simulink library "mbd_s32k11_ec_toolbox"  (Simulink 9.0)
settings: Solver=FixedStepDiscrete  StartTime=0.0  StopTime=10.0  FixedStep=0.1  RelTol=1e-3
InitFcn:
  | mbd_s32k11_consistency_checks(bdroot(gcs));
(part 2 of 2)

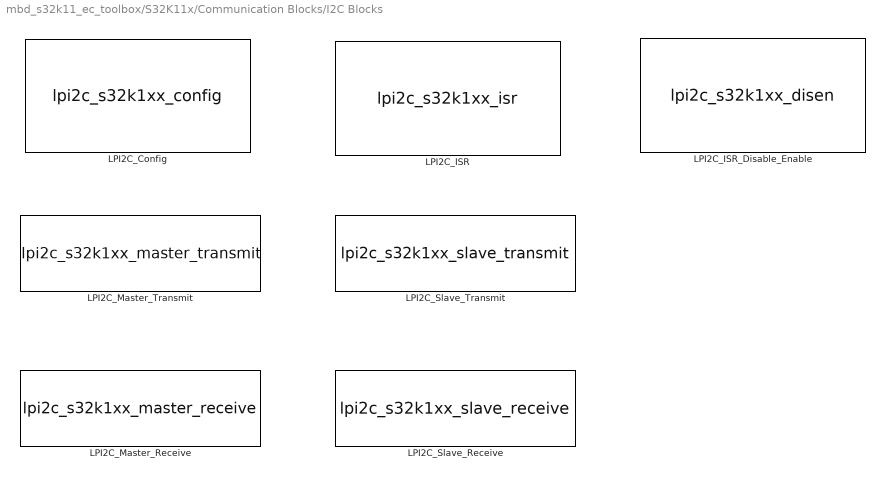
== system mbd_s32k11_ec_toolbox/S32K11x/Communication Blocks/I2C Blocks ==
  LPI2C_Config : S-Function  FunctionName=lpi2c_s32k1xx_config  SFunctionDeploymentMode=off  EnableBusSupport=off  mask(lpi2c_s32k1xx_config){instance=0, mode=Master, opmode=Standard (up to 100 kbit/s), bdr=100000, addr=1, is10bitaddr=off, sda=PTA2: [LPI2C0_SDA | LPI2C Data I/O], scl=PTA3: [LPI2C0_SCL | LPI2C Clock I/O]}
      mask prompts: opmode "Operating mode"; bdr "Baudrate, b/s"; addr "null"; is10bitaddr "10-bit address"
      mask help: This block allows to configure I2C module.
      mask init:
      | maskStr = mbd_s32k_lpi2c_config_string();
      | mbd_s32k_lpi2c_display_instances();
      | mbd_s32k_lpi2c_instance_callback(gcb);
      settings: NameChangeFcn=mbd_s32k_name_check(gcb);
      mask Help: web(fullfile(mbd_s32k11_block_help, 'lpi2c', 'lpi2c_config.html'));
      mask TypeOptions instance: 0
      mask Callback instance:
      | mbd_s32k_lpi2c_instance_callback(gcb);
      | mbd_s32k_lpi2c_display_instances();
      mask TypeOptions mode: Master | Slave
      mask Callback mode: mbd_s32k_lpi2c_mode_callback(gcb);
      mask TypeOptions opmode: Standard (up to 100 kbit/s)
      mask Callback bdr: mbd_s32k_lpi2c_check_bdr(gcb);
      mask TypeOptions sda: PTA2: [LPI2C0_SDA | LPI2C Data I/O] | PTB6: [LPI2C0_SDA | LPI2C Data I/O]
      mask TypeOptions scl: PTA3: [LPI2C0_SCL | LPI2C Clock I/O] | PTB7: [LPI2C0_SCL | LPI2C Clock I/O]
      mask Display: disp(maskStr);
  LPI2C_ISR : S-Function  FunctionName=lpi2c_s32k1xx_isr  SFunctionDeploymentMode=off  EnableBusSupport=off  mask(lpi2c_s32k1xx_isr){instance=0, mode=Master, rxreq=off, txreq=off, txempty=off, rxfull=off, stop=off, masterendtransfer=off, mastertx=off, masterrx=off, masterfifoerr=off, masterarblost=off, masternack=off}
      mask prompts: rxreq "I2C_SLAVE_EVENT_RX_REQ"; txreq "I2C_SLAVE_EVENT_TX_REQ"; txempty "I2C_SLAVE_EVENT_TX_EMPTY"; rxfull "I2C_SLAVE_EVENT_RX_FULL"; stop "I2C_SLAVE_EVENT_STOP"; masterendtransfer "I2C_MASTER_EVENT_END_TRANSFER"; mastertx "LPI2C_MASTER_EVENT_TX"; masterrx "LPI2C_MASTER_EVENT_RX"; masterfifoerr "LPI2C_MASTER_EVENT_FIFO_ERROR"; masterarblost "LPI2C_MASTER_EVENT_ARBITRATION_LOST"; masternack "LPI2C_MASTER_EVENT_NACK"
      mask help: This block allows to create routine for the LPI2C interrupts.
      mask init:
      | st = mbd_s32k_lpi2c_isr_tostring();
      | mbd_s32k_lpi2c_display_instances();
      settings: NameChangeFcn=mbd_s32k_name_check(gcb);
      mask Help: web(fullfile(mbd_s32k11_block_help, 'lpi2c', 'lpi2c_isr.html'));
      mask TypeOptions instance: 0
      mask Callback instance: mbd_s32k_lpi2c_display_instances();
      mask TypeOptions mode: Master | Slave
      mask Callback mode: mbd_s32k_lpi2c_isr_mode_ckb(gcb);
      mask Display:
      | disp(st);
      | port_label('output', 1, 'Trigger')
  LPI2C_ISR_Disable_Enable : S-Function  FunctionName=lpi2c_s32k1xx_disen  SFunctionDeploymentMode=off  EnableBusSupport=off  mask(lpi2c_s32k1xx_disen){instance=0, m_tdie=off, m_rdie=off, m_epie=off, m_sdie=off, m_ndie=off, m_alie=off, m_feie=off, s_tdie=off, s_rdie=off, s_rsie=off, s_sdie=off, s_beie=off, s_feie=off, upd=1}
      mask prompts: m_tdie "Transmit Data"; m_rdie "Receive Data"; m_epie "End Packet"; m_sdie "STOP Detect"; m_ndie "NACK Detect"; m_alie "Arbitration Lost"; m_feie "FIFO Error"; s_tdie "Transmit Data"; s_rdie "Receive Data"; s_rsie "Repeated Start"; s_sdie "STOP Detect"; s_beie "Bit Error"; s_feie "FIFO Error"
      mask help: This block allows to Enable/Disable I2C ISR routine.
      mask init:
      | mbd_s32k_lpi2c_display_instances();
      | 
      | eol = sprintf('\n');
      | st = ['LPI2C', get_param(gcb, 'instance')];
      | fields = get_param(gcb, 'MaskPrompts');
      | vis = get_param(gcb, 'MaskVisibilities');
      | vals = get_param(gcb, 'MaskValues');
      | 
      | for i = 2 : length(fields) - 1
      |     if (strcmp(vis{i}, 'on'))
      |         s = [eol, fields{i}, ': ', vals{i}];
      |         st = [st, s];
      |     end
      | end
      settings: NameChangeFcn=mbd_s32k_name_check(gcb);
      mask Help: web(fullfile(mbd_s32k11_block_help, 'lpi2c', 'lpi2c_disen.html'));
      mask TypeOptions instance: 0
      mask Callback instance: mbd_s32k_lpi2c_display_instances();
      mask Display: disp(st);
  LPI2C_Master_Receive : S-Function  FunctionName=lpi2c_s32k1xx_master_receive  SFunctionDeploymentMode=off  EnableBusSupport=off  mask(lpi2c_master_receive){instance=0, xfermode=Blocking, Timeout=50, is10bit=off}
      mask prompts: xfermode "Transfer mode"; Timeout "Timeout (ms)"; is10bit "10-bit address"
      mask help: This block allows the master to request data from slave.
      mask init:
      | maskStr = 'LPI2C Master Receive';
      | mbd_s32k_lpi2c_display_instances();
      settings: NameChangeFcn=mbd_s32k_name_check(gcb);
      mask Help: web(fullfile(mbd_s32k11_block_help, 'lpi2c', 'lpi2c_master_receive.html'));
      mask TypeOptions instance: 0
      mask Callback instance: mbd_s32k_lpi2c_display_instances();
      mask TypeOptions xfermode: Blocking | Non blocking
      mask Callback xfermode: mbd_s32k_lpi2c_xfer_mode_cbk()
      mask Display:
      | port_label('output', 1, 'Data');
      | port_label('input', 1, 'Address');
      | port_label('input', 2, 'SendStop');
      | port_label('input', 3, 'Length');
      | disp(maskStr);
  LPI2C_Master_Transmit : S-Function  FunctionName=lpi2c_s32k1xx_master_transmit  SFunctionDeploymentMode=off  EnableBusSupport=off  mask(lpi2c_master_transmit){instance=0, xfermode=Blocking, Timeout=50, is10bit=off}
      mask prompts: xfermode "Transfer mode"; Timeout "Timeout (ms)"; is10bit "10-bit address"
      mask help: This block allows the master to transmit data to the slave.
      mask init:
      | maskStr = 'LPI2C Master Transmit';
      | mbd_s32k_lpi2c_display_instances();
      settings: NameChangeFcn=mbd_s32k_name_check(gcb);
      mask Help: web(fullfile(mbd_s32k11_block_help, 'lpi2c', 'lpi2c_master_transmit.html'));
      mask TypeOptions instance: 0
      mask Callback instance: mbd_s32k_lpi2c_display_instances();
      mask TypeOptions xfermode: Blocking | Non blocking
      mask Callback xfermode: mbd_s32k_lpi2c_xfer_mode_cbk()
      mask Display:
      | port_label('input', 1, 'Data');
      | port_label('input', 2, 'SendStop');
      | port_label('input', 3, 'Address');
      | disp(maskStr);
  LPI2C_Slave_Receive : S-Function  FunctionName=lpi2c_s32k1xx_slave_receive  SFunctionDeploymentMode=off  EnableBusSupport=off  mask(lpi2c_slave_receive){instance=0, xfermode=Blocking, Timeout=50, is10bit=off}
      mask prompts: xfermode "Transfer mode"; Timeout "Timeout (ms)"; is10bit "10-bit address"
      mask help: This block allows the slave to receive data from master.
      mask init:
      | maskStr = 'LPI2C Slave Receive';
      | mbd_s32k_lpi2c_display_instances();
      settings: NameChangeFcn=mbd_s32k_name_check(gcb);
      mask Help: web(fullfile(mbd_s32k11_block_help, 'lpi2c', 'lpi2c_slave_receive.html'));
      mask TypeOptions instance: 0
      mask Callback instance: mbd_s32k_lpi2c_display_instances();
      mask TypeOptions xfermode: Blocking | Non blocking
      mask Callback xfermode: mbd_s32k_lpi2c_xfer_mode_cbk()
      mask Display:
      | port_label('output', 1, 'Data');
      | port_label('input', 1, 'Address');
      | port_label('input', 2, 'Length');
      | disp(maskStr);
  LPI2C_Slave_Transmit : S-Function  FunctionName=lpi2c_s32k1xx_slave_transmit  SFunctionDeploymentMode=off  EnableBusSupport=off  mask(lpi2c_slave_transmit){instance=0, xfermode=Blocking, Timeout=50, is10bit=off}
      mask prompts: xfermode "Transfer mode"; Timeout "Timeout (ms)"; is10bit "10-bit address"
      mask help: This block allows the slave to respond to master request for data.
      mask init:
      | maskStr = 'LPI2C Slave Transmit';
      | mbd_s32k_lpi2c_display_instances();
      settings: NameChangeFcn=mbd_s32k_name_check(gcb);
      mask Help: web(fullfile(mbd_s32k11_block_help, 'lpi2c', 'lpi2c_slave_transmit.html'));
      mask TypeOptions instance: 0
      mask Callback instance: mbd_s32k_lpi2c_display_instances();
      mask TypeOptions xfermode: Blocking | Non blocking
      mask Callback xfermode: mbd_s32k_lpi2c_xfer_mode_cbk()
      mask Display:
      | port_label('input', 1, 'Data');
      | port_label('input', 2, 'Address');
      | disp(maskStr);

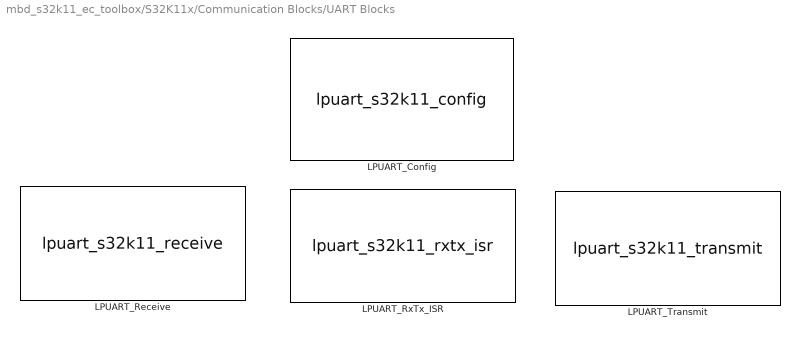
== system mbd_s32k11_ec_toolbox/S32K11x/Communication Blocks/UART Blocks ==
  LPUART_Config : S-Function  FunctionName=lpuart_s32k11_config  SFunctionDeploymentMode=off  EnableBusSupport=off  mask(lpuart_s32k11_config){instance=0, baudrate=115200, databits=8, parity=None, sbns=1, bothedge=rising edge, rxinv=off, txinv=off, show_adv_opts=off, brk13=10 - 13 bit times, lbkde=10 - 13 bit times, rx=PTA2: [LPUART0_RX | Receive], tx=PTA3: [LPUART0_TX | Transmit], cts=PTA0: [LPUART0_CTS | Clear To Send (bar)], rts=PTA1: [LPUART0_RTS | Request To Send]}
      mask prompts: instance "LPUART"; baudrate "Baud rate"; databits "Data bits"; parity "Parity mode"; sbns "Stop bit number select"; bothedge "Both edge sampling"; rxinv "Receive data inversion"; txinv "Transmit data inversion"; show_adv_opts "Show advanced options"; brk13 "Transmit break character length"; lbkde "Receive break character detection length"
      mask help: This block allows to configure LPUART module.
      mask init:
      | maskStr = mbd_s32k_lpuart_config_init();
      | mbd_s32k_lpuart_display_instances();
      | mbd_s32k_lpuart_instance_callback(gcb);
      settings: NameChangeFcn=mbd_s32k_name_check(gcb);
      mask Help: web(fullfile(mbd_s32k11_block_help, 'lpuart', 'lpuart_config.html'));
      mask TypeOptions instance: 0 | 1
      mask Callback instance:
      | mbd_s32k_lpuart_instance_callback(gcb);
      | mbd_s32k_lpuart_display_instances();
      mask TypeOptions baudrate: 1200 | 2400 | 4800 | 9600 | 14400 | 19200 | 38400 | 56000 | 57600 | 115200 | 128000 | 256000
      mask TypeOptions databits: 8 | 9 | 10
      mask TypeOptions parity: None | Even | Odd
      mask TypeOptions sbns: 1 | 2
      mask TypeOptions bothedge: rising edge | rising and falling edges
      mask Callback show_adv_opts: mbd_s32k_lpuart_config_cbk()
      mask TypeOptions brk13: 10 - 13 bit times | 13 - 16 bit times
      mask TypeOptions lbkde: 10 - 13 bit times | 13 - 16 bit times
      mask TypeOptions rx: PTA2: [LPUART0_RX | Receive] | PTB0: [LPUART0_RX | Receive] | PTC2: [LPUART0_RX | Receive]
      mask TypeOptions tx: PTA3: [LPUART0_TX | Transmit] | PTB1: [LPUART0_TX | Transmit] | PTC3: [LPUART0_TX | Transmit]
      mask TypeOptions cts: PTA0: [LPUART0_CTS | Clear To Send (bar)] | PTC8: [LPUART0_CTS | Clear To Send (bar)]
      mask TypeOptions rts: PTA1: [LPUART0_RTS | Request To Send] | PTC9: [LPUART0_RTS | Request To Send]
      mask Display: disp(maskStr);
  LPUART_Receive : S-Function  FunctionName=lpuart_s32k11_receive  SFunctionDeploymentMode=off  EnableBusSupport=off  mask(lpuart_s32k11_receive){instance=0}
      mask prompts: instance "LPUART"
      mask help: This block allows to read data from LPUART.
      mask init:
      | mbd_s32k_lpuart_display_instances();
      settings: NameChangeFcn=mbd_s32k_name_check(gcb);
      mask Help: web(fullfile(mbd_s32k11_block_help, 'lpuart', 'lpuart_receive.html'));
      mask TypeOptions instance: 0 | 1
      mask Callback instance: mbd_s32k_lpuart_display_instances();
      mask Display:
      | disp(['LPUART', get_param(gcb, 'instance')]);
      | port_label('output',1,'data');
      | port_label('input',1,'size');
  LPUART_RxTx_ISR : S-Function  FunctionName=lpuart_s32k11_rxtx_isr  Parameters=out_array  SFunctionDeploymentMode=off  EnableBusSupport=off  mask(lpuart_s32k11_rxtx_isr){instance=0, prio=0, tie=off, tcie=off, rie=off, ilie=off}
      mask prompts: instance "LPUART"; prio "ISR Priority"; tie "Transmit buffer empty"; tcie "End of transfer"; rie "Receiver buffer full"; ilie "Error event"
      mask help: This block allows to create receive/transmit ISR routine for the LPUART module.
      mask init:
      | mbd_s32k_lpuart_display_instances();
      | [out_struct, out_array] = mbd_s32k_lpuart_isr_info(gcb);
      | maskStr = mbd_s32k_lpuart_isr_string();
      settings: NameChangeFcn=mbd_s32k_name_check(gcb);
      mask Help: web(fullfile(mbd_s32k11_block_help, 'lpuart', 'lpuart_rxtx_isr.html'));
      mask TypeOptions instance: 0 | 1
      mask Callback instance: mbd_s32k_lpuart_display_instances();
      mask TypeOptions prio: 0 | 1 | 2 | 3 | 4 | 5 | 6 | 7 | 8 | 9 | 10 | 11 | 12 | 13 | 14 | 15
      mask Display:
      | port_label('output',1,'Trigger')
      | port_label('output',2,'Status')
      | disp(maskStr);
  LPUART_Transmit : S-Function  FunctionName=lpuart_s32k11_transmit  SFunctionDeploymentMode=off  EnableBusSupport=off  mask(lpuart_s32k11_transmit){instance=0}
      mask prompts: instance "LPUART"
      mask help: This block allows to transmit data via LPUART.
      mask init:
      | mbd_s32k_lpuart_display_instances();
      settings: NameChangeFcn=mbd_s32k_name_check(gcb);
      mask Help: web(fullfile(mbd_s32k11_block_help, 'lpuart', 'lpuart_transmit.html'));
      mask TypeOptions instance: 0 | 1
      mask Callback instance: mbd_s32k_lpuart_display_instances();
      mask Display:
      | disp(['LPUART', get_param(gcb, 'instance')]);
      | port_label('input',1,'data')

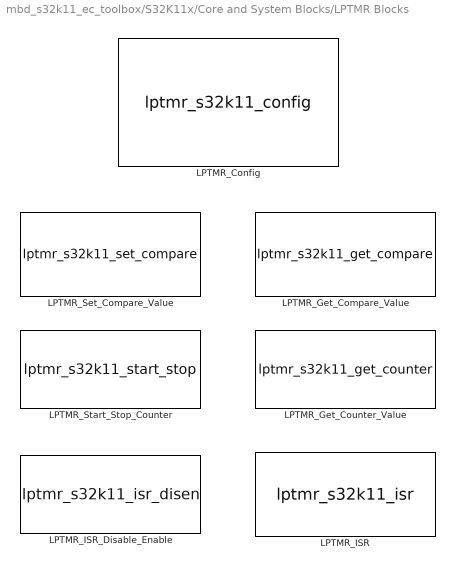
== system mbd_s32k11_ec_toolbox/S32K11x/Core and System Blocks/LPTMR Blocks ==
  LPTMR_Config : S-Function  FunctionName=lptmr_s32k11_config  SFunctionDeploymentMode=off  EnableBusSupport=off  mask(lptmr_s32k11_config){work_mode=Time Counter mode, compare_value=1, compare_value_units=Ticks, pin_select=Count pulses from pin alternative 2, pin_polarity=Count pulse on rising edge, pin_trgmux_source=Trigger function is disabled, show_adv_opts=off, input_clock=SIRC DIV2 clock, prescaler=Timer mode: prescaler 2, Glitch filter mode: invalid, bypass_prescaler=off, free_run=off, start_counter=on, enable_isr=on}
      mask prompts: work_mode "Mode Select"; compare_value "Compare Value"; compare_value_units "Compare Value Units"; pin_select "Pin Select"; pin_polarity "Pin Polarity"; pin_trgmux_source "TRGMUX Source"; show_adv_opts "Show advanced options"; input_clock "Prescaler Clock Select"; prescaler "Prescale Value"; bypass_prescaler "Prescaler Bypass"; free_run "Timer Free-Running Counter"; start_counter "Start  LPTMR counter immediatly after initialization"; enable_isr "Enable ISR immediatly after initialization"
      mask help: This block allows the user to configure the LPTMR module.
      mask init:
      | maskStr = mbd_s32k_lptmr_init();
      | 
      | set_param(gcb, 'MaskDisplay', ['disp(maskStr);']);
      settings: NameChangeFcn=mbd_s32k_name_check(gcb);
      mask Help: web(fullfile(mbd_s32k11_block_help, 'lptmr', 'lptmr_config.html'));
      mask TypeOptions work_mode: Time Counter mode | Pulse Counter mode
      mask Callback work_mode: mbd_s32k_lptmr_config_cbk('mode')
      mask TypeOptions compare_value_units: Ticks | Microseconds
      mask Callback compare_value_units: mbd_s32k_lptmr_config_cbk('units')
      mask TypeOptions pin_select: Count pulses from pin alternative 2 | Count pulses from pin alternative 3 | Count pulses from TRGMUX trigger
      mask Callback pin_select: mbd_s32k_lptmr_config_cbk('trgmux')
      mask TypeOptions pin_polarity: Count pulse on rising edge | Count pulse on falling edge
      mask TypeOptions pin_trgmux_source: Trigger function is disabled | Trigger MUX input 0 | Trigger MUX input 1 | Trigger MUX input 2 | Trigger MUX input 3 | Trigger MUX input 4 | Trigger MUX input 5 | Trigger MUX input 6 | Trigger MUX input 7 | Trigger MUX input 8 | Trigger MUX input 9 | Trigger MUX input 10 | Trigger MUX input 11 | CMP0 Output | LPIT Channel 0 | LPIT Channel 1 | LPIT Channel 2 | LPIT Channel 3 | LPTMR0 Trigger | FTM0 Internal Trigger | FTM0 External Trigger | FTM1 Internal Trigger | FTM1 External Trigger | FTM2 Internal Trigger | FTM2 External Trigger | FTM3 Internal Trigger | FTM3 External Trigger | ADC0_COCOA | ADC0_COCOB | ADC1_COCOA | ADC1_COCOB | PDB0 Channel 0 Trigger | PDB0 Pulse out | PDB1 Channel 0 Trigger | PDB1 Pulse out | RTC Alarm | RTC Seconds Counter | Flex IO Trigger 0 | Flex IO Trigger 1 | Flex IO Trigger 2 | Flex IO Trigger 3 | LPUART0 RX Data | LPUART0 TX Data | LPUART0 RX Idle | LPUART1 RX Data | LPUART1 TX Data | LPUART1 RX Idle | LPI2C0 Master Stop | LPI2C0 Slave Stop | LPI2C1 Master Stop | LPI2C1 Slave Stop | LPSPI0 Frame | LPSPI0 RX Data | LPSPI1 Frame | LPSPI1 RX Data | SIM Software Trigger
      mask Callback show_adv_opts: mbd_s32k_lptmr_config_cbk('show_adv_opts')
      mask TypeOptions input_clock: SIRC DIV2 clock | 1kHz LPO clock | RTC clock | PCC configured clock
      mask TypeOptions prescaler: Timer mode: prescaler 2, Glitch filter mode: invalid | Timer mode: prescaler 4, Glitch filter mode: 2 clocks | Timer mode: prescaler 8, Glitch filter mode: 4 clocks | Timer mode: prescaler 16, Glitch filter mode: 8 clocks | Timer mode: prescaler 32, Glitch filter mode: 16 clocks | Timer mode: prescaler 64, Glitch filter mode: 32 clocks | Timer mode: prescaler 128, Glitch filter mode: 64 clocks | Timer mode: prescaler 256, Glitch filter mode: 128 clocks | Timer mode: prescaler 512, Glitch filter mode: 256 clocks | Timer mode: prescaler 1024, Glitch filter mode: 512 clocks | Timer mode: prescaler 2048, Glitch filter mode: 1024 clocks | Timer mode: prescaler 4096, Glitch filter mode: 2048 clocks | Timer mode: prescaler 8192, Glitch filter mode: 4096 clocks | Timer mode: prescaler 16384, Glitch filter mode: 8192 clocks | Timer mode: prescaler 32768, Glitch filter mode: 16384 clocks | Timer mode: prescaler 65536, Glitch filter mode: 32768 clocks
      mask Callback bypass_prescaler: mbd_s32k_lptmr_config_cbk('prescaler')
      mask DialogControl timer_config_group Prompt: Timer configuration
      mask DialogControl source_config_group Prompt: Source configuration
      mask DialogControl prescaler_config_group Prompt: Prescaler configuration
      mask Display: disp(maskStr);
  LPTMR_Get_Compare_Value : S-Function  FunctionName=lptmr_s32k11_get_compare  Parameters=sFuncParams  SFunctionDeploymentMode=off  EnableBusSupport=off  mask(lptmr_s32k11_get_compare){compare_value_units=Ticks}
      mask prompts: compare_value_units "Compare Value Units"
      mask help: This block allows the user to get the compare value in counter tick units or microseconds, for LPTMR.
      mask init:
      | [maskStr ports sFuncParams] = mbd_s32k_lptmr_get_compare();
      | 
      | set_param(gcb, 'MaskDisplay', ['disp(maskStr);' ' ' ports]);
      settings: NameChangeFcn=mbd_s32k_name_check(gcb);
      mask Help: web(fullfile(mbd_s32k11_block_help, 'lptmr', 'lptmr_get_compare.html'));
      mask TypeOptions compare_value_units: Ticks | Microseconds
      mask Display: disp(maskStr); port_label('output', 1, 'Compare Value')
  LPTMR_Get_Counter_Value : S-Function  FunctionName=lptmr_s32k11_get_counter  SFunctionDeploymentMode=off  EnableBusSupport=off  mask(lptmr_s32k11_get_counter){}
      mask help: This block allows the user to get the current counter value in counter ticks units, for LPTMR.
      mask init:
      | [maskStr ports] = mbd_s32k_lptmr_get_counter();
      | 
      | set_param(gcb, 'MaskDisplay', ['disp(maskStr);' ' ' ports]);
      settings: NameChangeFcn=mbd_s32k_name_check(gcb);
      mask Help: web(fullfile(mbd_s32k11_block_help, 'lptmr', 'lptmr_get_counter.html'));
      mask Display: disp(maskStr); port_label('output', 1, 'Counter Value')
  LPTMR_ISR : S-Function  FunctionName=lptmr_s32k11_isr  SFunctionDeploymentMode=off  EnableBusSupport=off  mask(lptmr_s32k11_isr){}
      mask help: This block allows to call user function on LPTMR interrupt.
      settings: NameChangeFcn=mbd_s32k_name_check(gcb);
      mask Help: web(fullfile(mbd_s32k11_block_help, 'lptmr', 'lptmr_isr.html'));
      mask Display: disp('LPTMR ISR')
  LPTMR_ISR_Disable_Enable : S-Function  FunctionName=lptmr_s32k11_isr_disen  SFunctionDeploymentMode=off  EnableBusSupport=off  mask(lptmr_s32k11_isr_disen){set_action=Enable}
      mask prompts: set_action "Action"
      mask help: This block allows the user to enable or disable the LPTMR.
      mask init:
      | maskStr = mbd_s32k_lptmr_isr_disen();
      | 
      | set_param(gcb, 'MaskDisplay', 'disp(maskStr);');
      settings: NameChangeFcn=mbd_s32k_name_check(gcb);
      mask Help: web(fullfile(mbd_s32k11_block_help, 'lptmr', 'lptmr_isr_disable_enable.html'));
      mask TypeOptions set_action: Enable | Disable
      mask Display: disp(maskStr);
  LPTMR_Set_Compare_Value : S-Function  FunctionName=lptmr_s32k11_set_compare  Parameters=sFuncParams  SFunctionDeploymentMode=off  EnableBusSupport=off  mask(lptmr_s32k11_set_compare){compare_value_units=Microseconds}
      mask prompts: compare_value_units "Compare Value Units"
      mask help: This block allows the user to set the compare value in counter tick units or microsenconds, for LPTMR.
      mask init:
      | [maskStr ports sFuncParams] = mbd_s32k_lptmr_set_compare();
      | 
      | set_param(gcb, 'MaskDisplay', ['disp(maskStr);' ' ' ports]);
      settings: NameChangeFcn=mbd_s32k_name_check(gcb);
      mask Help: web(fullfile(mbd_s32k11_block_help, 'lptmr', 'lptmr_set_compare.html'));
      mask TypeOptions compare_value_units: Ticks | Microseconds
      mask Display: disp(maskStr); port_label('input', 1, 'Compare Value')
  LPTMR_Start_Stop_Counter : S-Function  FunctionName=lptmr_s32k11_start_stop  SFunctionDeploymentMode=off  EnableBusSupport=off  mask(lptmr_s32k11_start_stop){set_action=Start}
      mask prompts: set_action "Action"
      mask help: This block allows the user to start or stop the LPTMR.
      mask init:
      | maskStr = mbd_s32k_lptmr_start_stop();
      | 
      | set_param(gcb, 'MaskDisplay', 'disp(maskStr);');
      settings: NameChangeFcn=mbd_s32k_name_check(gcb);
      mask Help: web(fullfile(mbd_s32k11_block_help, 'lptmr', 'lptmr_start_stop.html'));
      mask TypeOptions set_action: Start | Stop
      mask Display: disp(maskStr);

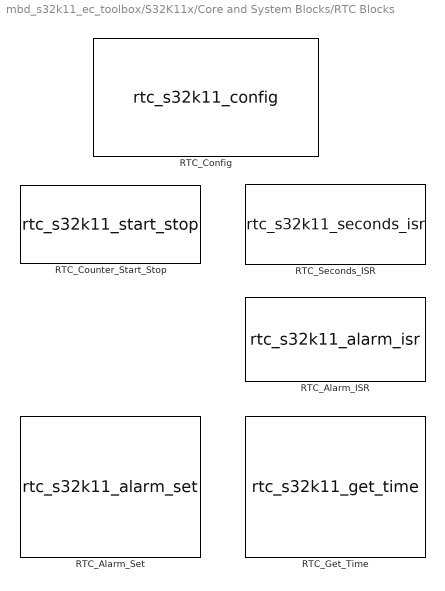
== system mbd_s32k11_ec_toolbox/S32K11x/Core and System Blocks/RTC Blocks ==
  RTC_Alarm_ISR : S-Function  FunctionName=rtc_s32k11_alarm_isr  SFunctionDeploymentMode=off  EnableBusSupport=off  mask(rtc_s32k11_alarm_isr){}
      mask help: This block allows to call user function on RTC interrupt.
      settings: NameChangeFcn=mbd_s32k_name_check(gcb);
      mask Help: web(fullfile(mbd_s32k11_block_help, 'rtc', 'rtc_alarm_isr.html'));
      mask Display: disp('RTC Alarm ISR')
  RTC_Alarm_Set : S-Function  FunctionName=rtc_s32k11_alarm_set  Parameters=sFuncParams  SFunctionDeploymentMode=off  EnableBusSupport=off  mask(rtc_s32k11_alarm_set){inputs_enable=off, date_day=1, date_month=1, date_year=1970, time_hour=0, time_min=0, time_sec=0, show_adv_opts=off, repeat=off, interval=0, forever=on, repeats=0}
      mask prompts: inputs_enable "Date/Time as inputs"; date_day "Date (dd/mm/yy)"; time_hour "Time (hh:mm::ss)"; show_adv_opts "Show advanced options"; interval "Repeat interval (seconds)"; forever "Repeat forever"; repeats "Number of repeats"
      mask help: This block allows the user to set an alarm.
      mask init:
      | [st,labels] = mbd_s32k_rtc_alarm_set_init();
      | sFuncParams = [inputs_enable]';
      | set_param(gcb, 'MaskDisplay', labels);
      settings: NameChangeFcn=mbd_s32k_name_check(gcb);
      mask Help: web(fullfile(mbd_s32k11_block_help, 'rtc', 'rtc_alarm_set.html'));
      mask Callback inputs_enable: mbd_s32k_rtc_alarm_set_cbk('inputs_enable')
      mask Callback show_adv_opts: mbd_s32k_rtc_alarm_set_cbk('show_adv_opts')
      mask Callback repeat: mbd_s32k_rtc_alarm_set_cbk('repeat_enable')
      mask Callback forever: mbd_s32k_rtc_alarm_set_cbk('repeat_forever')
      mask Display: disp(st);
  RTC_Config : S-Function  FunctionName=rtc_s32k11_config  SFunctionDeploymentMode=off  EnableBusSupport=off  mask(rtc_s32k11_config){date_day=1, date_month=1, date_year=1970, time_hour=0, time_min=0, time_sec=0, show_adv_opts=on, clock_input=1KHz LPO, clock_output=Disabled, comp_state=on, comp_value=0, comp_interval=0, state_update=off, state_w_access=off, state_read_only=off, start_counter=on}
      mask prompts: date_day "Date"; time_hour "Time"; show_adv_opts "Show advanced options"; clock_input "Input Clock"; clock_output "Clock Out"; comp_state "Compensation"; comp_value "Compensation value            [-127,128]"; comp_interval "Compensation interval              [0,255]"; state_update "Update"; state_w_access "Non-supervisor write access"; state_read_only "Read-only"; start_counter "Start RTC counter immediatly after initialization"
      mask help: This block allows the user to configure the RTC module.
      mask init:
      | maskStr = mbd_s32k_rtc_config_init();
      | 
      | set_param(gcb, 'MaskDisplay', ['disp(maskStr);']);
      settings: NameChangeFcn=mbd_s32k_name_check(gcb);
      mask Help: web(fullfile(mbd_s32k11_block_help, 'rtc', 'rtc_config.html'));
      mask Callback show_adv_opts: mbd_s32k_rtc_config_cbk('show_adv_opts')
      mask TypeOptions clock_input: 32KHz crystal | 1KHz LPO
      mask TypeOptions clock_output: Disabled | Prescaler output | 32KHz clock
      mask Callback comp_state: mbd_s32k_rtc_config_cbk('compensation')
      mask Callback comp_interval: mbd_s32k_rtc_config_cbk('comp_value')
      mask DialogControl time_config_group Prompt: Time configuration
      mask DialogControl time_config_group_copy Prompt: Time configuration
      mask Display: disp(maskStr);
  RTC_Counter_Start_Stop : S-Function  FunctionName=rtc_s32k11_start_stop  SFunctionDeploymentMode=off  EnableBusSupport=off  mask(rtc_s32k11_counter_start_stop){set_action=Start}
      mask prompts: set_action "Action"
      mask help: This block allows the user to start or stop the RTC counter.
      mask init:
      | maskStr = mbd_s32k_rtc_start_stop();
      | set_param(gcb, 'MaskDisplay', 'disp(maskStr);');
      settings: NameChangeFcn=mbd_s32k_name_check(gcb);
      mask Help: web(fullfile(mbd_s32k11_block_help, 'rtc', 'rtc_s32k14_counter_start_stop.html'));
      mask TypeOptions set_action: Start | Stop
      mask Display: disp(maskStr);
  RTC_Get_Time : S-Function  FunctionName=rtc_s32k11_get_time  SFunctionDeploymentMode=off  EnableBusSupport=off  mask(rtc_s32k11_get_time){}
      mask help: This block returns the time to the user.
      mask init:
      | [st,labels] = mbd_s32k_rtc_get_time_init();
      | set_param(gcb, 'MaskDisplay', labels);
      settings: NameChangeFcn=mbd_s32k_name_check(gcb);
      mask Help: web(fullfile(mbd_s32k11_block_help, 'rtc', 'rtc_get_time.html'));
      mask Display:
      | port_label('output', 1, 'Year')
      | port_label('output', 2, 'Month')
      | port_label('output', 3, 'Day')
      | port_label('output', 4, 'Hours')
      | port_label('output', 5, 'Minutes')
      | port_label('output', 6, 'Seconds')
      | disp(st);
  RTC_Seconds_ISR : S-Function  FunctionName=rtc_s32k11_seconds_isr  SFunctionDeploymentMode=off  EnableBusSupport=off  mask(rtc_s32k11_seconds_isr){sec_irq_freq=1Hz}
      mask prompts: sec_irq_freq "Frequency"
      mask help: This block allows to call user function on RTC interrupt.
      mask init:
      | maskStr = mbd_s32k_rtc_seconds_isr_init();
      | 
      | set_param(gcb, 'MaskDisplay', ['disp(maskStr);']);
      settings: NameChangeFcn=mbd_s32k_name_check(gcb);
      mask Help: web(fullfile(mbd_s32k11_block_help, 'rtc', 'rtc_alarm_seconds_isr.html'));
      mask TypeOptions sec_irq_freq: 1Hz | 2Hz | 4Hz | 8Hz | 16Hz | 32Hz | 64Hz | 128Hz
      mask DialogControl Container3 Prompt: General
      mask Display: disp(maskStr);

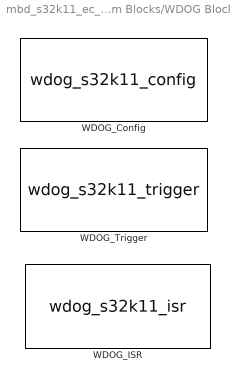
== system mbd_s32k11_ec_toolbox/S32K11x/Core and System Blocks/WDOG Blocks ==
  WDOG_Config : S-Function  FunctionName=wdog_s32k11_config  Parameters=sFuncParams  SFunctionDeploymentMode=off  EnableBusSupport=off  mask(wdog_s32k11_config){clk_source=SIRC clock, window_enable=off, window_value=2.000, window_value_unit=milliseconds, timeout_value=2.000, timeout_value_unit=seconds, prescaler_enable=on, update_enable=off, int_enable=on, show_adv_opts=off}
      mask prompts: clk_source "Clock source"; window_enable "Window enable"; window_value "Window value"; timeout_value "Timeout value"; prescaler_enable "Prescaler enable"; update_enable "Update enable"; int_enable "Interrupt enable"; show_adv_opts "Show advanced options"
      mask help: This block allows the user to configure the WDOG module.
      mask init:
      | maskStr = 'WDOG Config';
      | 
      | sFuncParams = [
      |     clk_source
      |     update_enable
      |     int_enable
      |     window_enable
      |     window_value
      |     window_value_unit
      |     timeout_value
      |     timeout_value_unit
      |     prescaler_enable];
      settings: NameChangeFcn=mbd_s32k_name_check(gcb);
      mask Help: web(fullfile(mbd_s32k11_block_help, 'wdog', 'wdog_config.html'));
      mask TypeOptions clk_source: Bus clock | LPO clock | SOSC clock | SIRC clock
      mask Callback clk_source: mbd_s32k_wdog_config_cbk('clk_source')
      mask Callback window_enable: mbd_s32k_wdog_config_cbk('window_enable')
      mask Callback window_value: mbd_s32k_wdog_config_cbk('window_value')
      mask TypeOptions window_value_unit: seconds | milliseconds | microseconds | clock cycles
      mask Callback window_value_unit: mbd_s32k_wdog_config_cbk('window_value_unit')
      mask Callback timeout_value: mbd_s32k_wdog_config_cbk('timeout_value')
      mask TypeOptions timeout_value_unit: seconds | milliseconds | microseconds | clock cycles
      mask Callback timeout_value_unit: mbd_s32k_wdog_config_cbk('timeout_value_unit')
      mask Callback prescaler_enable: mbd_s32k_wdog_config_cbk('prescaler_enable')
      mask Callback show_adv_opts: mbd_s32k_wdog_config_cbk('show_adv_opts')
      mask DialogControl GeneralTab Prompt: General
      mask DialogControl SourceClockFreqText Prompt: Source clock frequency: 8 MHz
      mask DialogControl WindowGroupbox Prompt: Window
      mask DialogControl TimeoutGroupbox Prompt: Timeout
      mask Display: disp(maskStr)
  WDOG_ISR : S-Function  FunctionName=wdog_s32k11_isr  SFunctionDeploymentMode=off  EnableBusSupport=off  mask(wdog_s32k11_isr){}
      mask help: This block allows to call user function on WDOG timeout interrupt.
      settings: NameChangeFcn=mbd_s32k_name_check(gcb);
      mask Help: web(fullfile(mbd_s32k11_block_help, 'wdog', 'wdog_isr.html'));
      mask Display: disp('WDOG ISR')
  WDOG_Trigger : S-Function  FunctionName=wdog_s32k11_trigger  SFunctionDeploymentMode=off  EnableBusSupport=off  mask(wdog_s32k11_trigger){}
      mask help: This block allows the user to refresh the WDOG counter.
      settings: NameChangeFcn=mbd_s32k_name_check(gcb);
      mask Help: web(fullfile(mbd_s32k11_block_help, 'wdog', 'wdog_trigger.html'));
      mask Display: disp('WDOG Trigger')

== system mbd_s32k11_ec_toolbox/S32K11x/Motor Control Blocks/CMP Blocks ==
  CMP_Config : S-Function  FunctionName=cmp_s32k11_config  SFunctionDeploymentMode=off  EnableBusSupport=off  mask(cmp_s32k11_config){instance=0, mode=Continuous, fpr=0, pmode=Low Speed, invt=off, cos=Set CMPO to equal COUT (filtered), ope=PTA4: [CMP0_OUT | Comparator Output trigger], filter_cnt=Disabled, offset=level 0, hystctr=level 0, inpsel=IN0, from the 8-bit DAC output, innsel=IN0, from the 8-bit DAC output, chn0=off, chn1=off, chn2=off, chn3=off, chn4=off, chn5=off, chn6=off, chn7=off, dacen=on, vrsel=Vin1, psel=PTA0: [CMP0_IN0 | Comparator Input Signal], msel=PTA1: [CMP0_IN1 | Comparator Input Signal], vosel=0, rre=off, fxmp=The Plus port is fixed, fxmxch=Channel 0, nsam=as soon as the active channel is scanned, mcuTargetUpdate=on}
      mask prompts: instance "CMP"; fpr "Filter Sample Period"; pmode "Power Mode Select"; invt "Comparator Invert"; cos "Comparator Output Select"; ope "Comparator Output Pin Enable"; filter_cnt "Filter Sample Count"; offset "Offset Control"; hystctr "Hysteresis Control"; inpsel "Selection of the input to the positive port"; innsel "Selection of the input to the negative port"; chn0 "Channel 0 input enable"; chn1 "Channel 1 input enable"; chn2 "Channel 2 input enable"; chn3 "Channel 3 input enable"; chn4 "Channel 4 input enable"; chn5 "Channel 5 input enable"; chn6 "Channel 6 input enable"; chn7 "Channel 7 input enable"; dacen "DAC Enable"; vrsel "Supply Voltage Reference Source Select"; psel "Plus Input MUX Control"; msel "Minus Input MUX Control"; vosel "DAC Output Voltage Select"; rre "Round-Robin Enable"; fxmp "Fixed MUX Port"; fxmxch "Fixed Channel Selection"; nsam "Number of Sample Clocks"
      mask help: This block allows to configure CMP module.
      mask init:
      | [maskStr] = mbd_s32k_cmp_config_init();
      | mbd_s32k_cmp_config_display();
      settings: NameChangeFcn=mbd_s32k_name_check(gcb);
      mask Help: web(fullfile(mbd_s32k11_block_help, 'cmp', 'cmp_config.html'));
      mask TypeOptions instance: 0
      mask TypeOptions mode: Continuous | Sampled Non-Filtered Int Clock | Sampled Non-Filtered Ext Clock | Sampled Filtered Int Clock | Sampled Filtered Ext Clock | Window | Windowed Resampled | Windowed Filtered
      mask Callback mode: mbd_s32k_cmp_config_cbk('mode');
      mask Callback fpr: mbd_s32k_cmp_config_cbk('fpr')
      mask TypeOptions pmode: Low Speed | High Speed
      mask TypeOptions cos: Set CMPO to equal COUT (filtered) | Set CMPO to equal COUTA (unfiltered)
      mask TypeOptions ope: PTA4: [CMP0_OUT | Comparator Output trigger]
      mask TypeOptions filter_cnt: Disabled | 1 consecutive sample must agree | 2 consecutive samples must agree | 3 consecutive samples must agree | 4 consecutive samples must agree | 5 consecutive samples must agree | 6 consecutive samples must agree | 7 consecutive samples must agree
      mask TypeOptions offset: level 0 | level 1
      mask TypeOptions hystctr: level 0 | level 1 | level 2 | level 3
      mask TypeOptions inpsel: IN0, from the 8-bit DAC output | IN1, from the analog 8-1 mux
      mask TypeOptions innsel: IN0, from the 8-bit DAC output | IN1, from the analog 8-1 mux
      mask TypeOptions vrsel: Vin1 | Vin2
      mask TypeOptions psel: PTA0: [CMP0_IN0 | Comparator Input Signal] | PTA1: [CMP0_IN1 | Comparator Input Signal] | PTC4: [CMP0_IN2 | Comparator Input Signal] | PTE8: [CMP0_IN3 | Comparator Input Signal] | PTC3: [CMP0_IN4 | Comparator Input Signal] | PTC2: [CMP0_IN5 | Comparator Input Signal]
      mask TypeOptions msel: PTA0: [CMP0_IN0 | Comparator Input Signal] | PTA1: [CMP0_IN1 | Comparator Input Signal] | PTC4: [CMP0_IN2 | Comparator Input Signal] | PTE8: [CMP0_IN3 | Comparator Input Signal] | PTC3: [CMP0_IN4 | Comparator Input Signal] | PTC2: [CMP0_IN5 | Comparator Input Signal]
      mask Callback vosel: mbd_s32k_cmp_config_cbk('vosel');
      mask TypeOptions fxmp: The Plus port is fixed | The Minus port is fixed
      mask TypeOptions fxmxch: Channel 0 | Channel 1 | Channel 2 | Channel 3 | Channel 4 | Channel 5
      mask TypeOptions nsam: as soon as the active channel is scanned | 1 round-robin clock cycle after the next cycle | 2 round-robin clock cycles after the next cycle | 3 round-robin clock cycles after the next cycle
      mask Display: disp(maskStr);
  CMP_ISR : S-Function  FunctionName=cmp_s32k11_isr  SFunctionDeploymentMode=off  EnableBusSupport=off  mask(cmp_s32k11_isr){instance=0, ier=off, ief=off, prio=0}
      mask prompts: instance "CMP"; ier "Rising ISR"; ief "Falling ISR"; prio "ISR Priority"
      mask help: This block allows to configure Comparator ISR routine.
      mask init:
      | [maskStr] = mbd_s32k_cmp_isr_init();
      settings: NameChangeFcn=mbd_s32k_name_check(gcb);
      mask Help: web(fullfile(mbd_s32k11_block_help, 'cmp', 'cmp_isr.html'));
      mask TypeOptions instance: 0
      mask TypeOptions prio: 0 | 1 | 2 | 3 | 4 | 5 | 6 | 7 | 8 | 9 | 10 | 11 | 12 | 13 | 14 | 15
      mask DialogControl ParameterTabVar0 Prompt: General
      mask Display:
      | disp(maskStr);
      | port_label('output',1,'trigger');
      | port_label('output',2,'CFR');
      | port_label('output',3,'CFF');
  CMP_ISR_Enable_Disable : S-Function  FunctionName=cmp_s32k11_isr_disen  SFunctionDeploymentMode=off  EnableBusSupport=off  mask(cmp_s32k11_control_isr_disen){instance=0, ier=off, ief=off}
      mask prompts: instance "CMP"; ier "Rising ISR"; ief "Falling ISR"
      mask help: This block enables or disables the interrupts for CMP block.
      mask init:
      | [maskStr] = mbd_s32k_cmp_isr_disen_init();
      settings: NameChangeFcn=mbd_s32k_name_check(gcb);
      mask Help: web(fullfile(mbd_s32k11_block_help, 'cmp', 'cmp_isr_disen.html'));
      mask TypeOptions instance: 0
      mask Display: disp(maskStr)
